simulink model "pendulum"  (R2021a)
settings: Solver=FixedStepAuto  StartTime=0.0  StopTime=20  FixedStep=0.001  MaxStep=0.001  RelTol=1e-3
undefined symbols (not defined in the file): d, g, l, omega_0, theta_0
libraries: simulink_extras x1
settings Model: Creator=lennartfuhrig  LastModifiedBy=lennartfuhrig

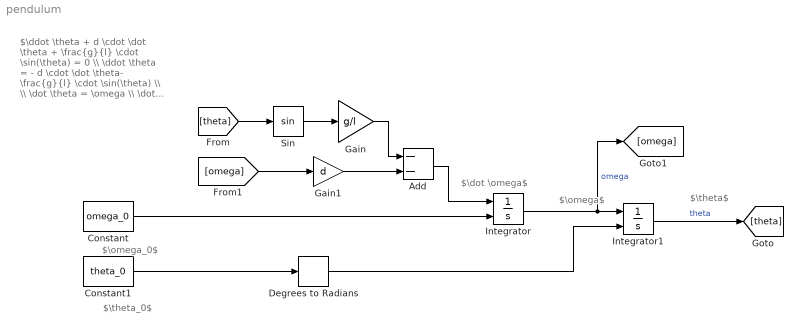
== system pendulum ==
  note: $\dot \omega$
  note: $\omega$
  note: $\theta$
  note: $\omega_0$
  note: $\theta_0$
  note: $\ddot \theta + d \cdot \dot \theta + \frac{g}{l} \cdot \sin(\theta) = 0 \\ \ddot \theta = - d \cdot \dot \theta- \frac{g}{l} \cdot \sin(\theta) \\ \\ \dot \theta = \omega \\ \dot \omega = - d \cdot \omega - \frac{g}{l} \cdot \sin(\theta)$
  Add : Sum  Inputs=--
  Constant : Constant  Value=omega_0
  Constant1 : Constant  Value=theta_0
  Degrees to Radians : simulink_extras/Transformations/Degrees to Radians
  Gain : Gain  Gain=g/l
  Gain1 : Gain  Gain=d
  Integrator : Integrator  InitialConditionSource=external
  Integrator1 : Integrator  InitialConditionSource=external
  Sin : Trigonometry
  wires:
  Integrator/1 -> [omega], Integrator1/1  "omega"
  Constant/1 -> Integrator/2
  Integrator1/1 -> [theta]  "theta"
  Sin/1 -> Gain/1
  [theta] -> Sin/1
  Add/1 -> Integrator/1
  Gain/1 -> Add/1
  Gain1/1 -> Add/2
  [omega] -> Gain1/1
  Constant1/1 -> Degrees to Radians/1
  Degrees to Radians/1 -> Integrator1/2
